simulink model "ObjectPixelCount"  (R2016a)
settings: Solver=VariableStepAuto  StartTime=0.0  StopTime=10.0  RelTol=1e-3
undefined symbols (not defined in the file): Rec, SDTV
libraries: visionsinks x3, visionconversions x2, visionsources x2
settings Model: Creator=YASARA  LastModifiedBy=YASARA

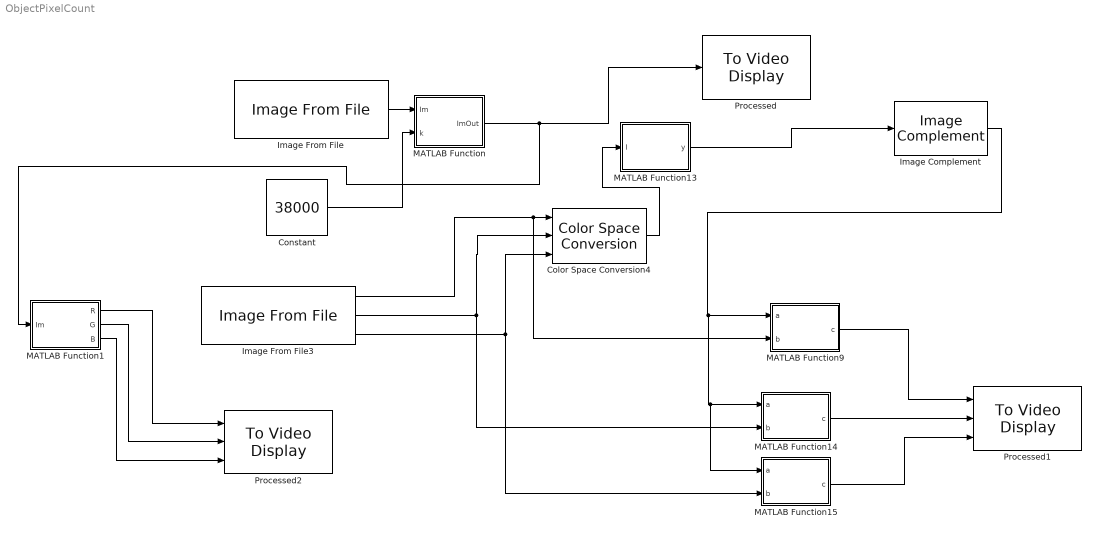
== system ObjectPixelCount ==
  Color Space Conversion4 : visionconversions/Color Space  Conversion  conversion=Obsolete  conversionActive=R'G'B' to intensity  wp_str=D65  rec=Rec. 601 (SDTV)  sys=1125/60/2:1  imagePorts=Separate color signals
  Constant : Constant  Value=38000  OutDataTypeStr=uint32  SampleTime=100000
  Image Complement : visionconversions/Image Complement
  Image From File : visionsources/Image From File  Tag=vipblks_nd  FileName=C:\Users\YASARA\Desktop\New folder (3)\Testing\OPA_OPA\Resolution1\DSC_1237.JPG  imagePorts=One multidimensional signal  Ts=100000  ImageDataType=Inherit from input image  Signed=on  WordLength=16  sdImageDataType=uint(8)  FractionLengthMode=User-defined  FractionLength=15  OutPortLabels=R|G|B
  Image From File3 : visionsources/Image From File  Tag=vipblks_nd  FileName=C:\Users\YASARA\Desktop\New folder (3)\Testing\OPA_OPA\Resolution1\DSC_1237.JPG  imagePorts=Separate color signals  Ts=1  ImageDataType=double  Signed=on  WordLength=16  sdImageDataType=uint(8)  FractionLengthMode=User-defined  FractionLength=15  OutPortLabels=R|G|B
  MATLAB Function : MATLAB Function  TreatAsAtomicUnit=on
  MATLAB Function1 : MATLAB Function  TreatAsAtomicUnit=on
  MATLAB Function13 : MATLAB Function  TreatAsAtomicUnit=on
  MATLAB Function14 : MATLAB Function  TreatAsAtomicUnit=on
  MATLAB Function15 : MATLAB Function  TreatAsAtomicUnit=on
  MATLAB Function9 : MATLAB Function  TreatAsAtomicUnit=on
  Processed : visionsinks/To Video Display  windowSizeMode=Normal  openAtMdlStart=on  fullScreen=off  videoWindowX=784  videoWindowY=165  saveWindowSize=off  videoWindowWidth=512  videoWindowHeight=384  inputColorFormat=RGB  inputType=Obsolete  imagePorts=One multidimensional signal  OutputDevice=On-screen video monitor  dataOrg=Column-major  isWindowOpen=off
  Processed1 : visionsinks/To Video Display  windowSizeMode=Normal  openAtMdlStart=on  fullScreen=off  videoWindowX=611  videoWindowY=290  saveWindowSize=off  videoWindowWidth=512  videoWindowHeight=384  inputColorFormat=RGB  inputType=Obsolete  imagePorts=Separate color signals  OutputDevice=On-screen video monitor  dataOrg=Column-major  isWindowOpen=off
  Processed2 : visionsinks/To Video Display  windowSizeMode=Normal  openAtMdlStart=on  fullScreen=off  videoWindowX=784  videoWindowY=165  saveWindowSize=off  videoWindowWidth=512  videoWindowHeight=384  inputColorFormat=RGB  inputType=Obsolete  imagePorts=Separate color signals  OutputDevice=On-screen video monitor  dataOrg=Column-major  isWindowOpen=off
  wires:
  Image From File/1 -> MATLAB Function/1(Im)
  MATLAB Function/1(ImOut) -> MATLAB Function1/1(Im), Processed/1
  Constant/1 -> MATLAB Function/2(k)
  Color Space Conversion4/1 -> MATLAB Function13/1(I)
  MATLAB Function9/1(c) -> Processed1/1
  MATLAB Function14/1(c) -> Processed1/2
  MATLAB Function15/1(c) -> Processed1/3
  Image From File3/1 -> MATLAB Function9/2(b), Color Space Conversion4/1
  Image From File3/2 -> Color Space Conversion4/2, MATLAB Function14/2(b)
  Image From File3/3 -> Color Space Conversion4/3, MATLAB Function15/2(b)
  MATLAB Function13/1(y) -> Image Complement/1
  Image Complement/1 -> MATLAB Function15/1(a), MATLAB Function14/1(a), MATLAB Function9/1(a)
  MATLAB Function1/1(R) -> Processed2/1
  MATLAB Function1/2(G) -> Processed2/2
  MATLAB Function1/3(B) -> Processed2/3

== matlab function ObjectPixelCount/MATLAB Function ==
  data: Im input; ImOut output; k input
function ImOut = fcn(Im,k)
I=rgb2gray(Im);
coder.extrinsic('graythresh');
coder.extrinsic('im2bw');
level = graythresh(I);
BW = im2bw(I,level);
L=double(I);
coder.extrinsic('bwlabeln');
NUM=1;
BW2=imcomplement(BW);
[L, NUM] = bwlabeln(BW2);
area=1;
n=1;
R1=Im(:,:,1);
R2=Im(:,:,1);
R3=Im(:,:,1);
AA=1;

for n=1:NUM
    [r, c] = find(L==n);
    if (length(r)>1000) && (length(c)>1000)
        AA=max(length(r),length(c));
        if AA<k
           R1(L==n)=0; 
           R2(L==n)=0;            
           R3(L==n)=0;
        end
    end
end
II=Im;
II=cat(3,R1,R2,R3);
ImOut=II;

== matlab function ObjectPixelCount/MATLAB Function14 ==
  data: a input; b input; c output
function c = fcn(a,b)
%#codegen
c=a.*b;
return

== matlab function ObjectPixelCount/MATLAB Function1 ==
  data: Im input; R output; G output; B output
function [R,G,B] = fcn(Im)

R=double(Im(:,:,1));
G=double(Im(:,:,2));
B=double(Im(:,:,3));

== matlab function ObjectPixelCount/MATLAB Function13 ==
  data: I input; y output
function y = fcn(I)
%#codegen
y=I;
 coder.extrinsic('graythresh');
level = graythresh(I);
BW = double(im2bw(I,level));
y = BW;

== matlab function ObjectPixelCount/MATLAB Function15 ==
  data: a input; b input; c output
function c = fcn(a,b)
%#codegen
c=a.*b;
return

== matlab function ObjectPixelCount/MATLAB Function9 ==
  data: a input; b input; c output
function c = fcn(a,b)
%#codegen
c=a.*b;
return
